simulink model "LAB4"  (R2025b)
settings: Solver=VariableStepAuto  StartTime=0.0  StopTime=20  RelTol=1e-3
libraries: simulink x1
settings Model: Creator=Wingshingsho  LastModifiedBy=Wingshingsho

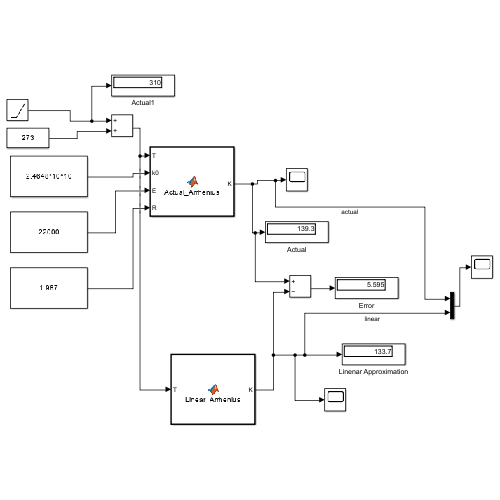
[thumbnail: Simulink's stored preview of the top-level diagram]
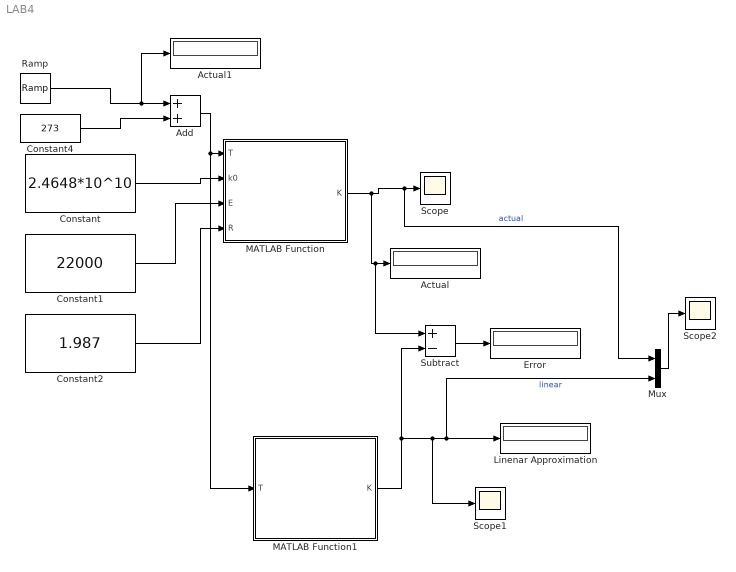
== system LAB4 ==
  Actual : Display
  Actual1 : Display
  Add : Sum
  Constant : Constant  Value=2.4648*10^10
  Constant1 : Constant  Value=22000
  Constant2 : Constant  Value=1.987
  Constant4 : Constant  Value=273
  Error : Display
  Linenar Approximation : Display
  MATLAB Function : MATLAB Function  TreatAsAtomicUnit=on
  MATLAB Function1 : MATLAB Function  TreatAsAtomicUnit=on
  Mux : Mux  Inputs=2
  Ramp : simulink/Sources/Ramp  slope=(310-290)/20  start=0  InitialOutput=290
  Scope : Scope
      settings: ActiveDisplayYMinimum=62.404399178444322  ActiveDisplayYMaximum=147.8382745404146
  Scope1 : Scope
      settings: ActiveDisplayYMinimum=-1  ActiveDisplayYMaximum=1
  Scope2 : Scope
      settings: ActiveDisplayYMinimum=57.175639124472795  ActiveDisplayYMaximum=148.41924787974477  DataLoggingVariableName=ScopeData2
  Subtract : Sum  Inputs=+-
  wires:
  Constant1/1 -> MATLAB Function/3(E)
  Constant/1 -> MATLAB Function/2(k0)
  Constant2/1 -> MATLAB Function/4(R)
  Constant4/1 -> Add/2
  Add/1 -> MATLAB Function1/1(T), MATLAB Function/1(T)
  MATLAB Function/1(K) -> Subtract/1, Actual/1, Mux/1, Scope/1  "actual"
  MATLAB Function1/1(K) -> Subtract/2, Scope1/1, Mux/2, Linenar Approximation/1  "linear"
  Subtract/1 -> Error/1
  Ramp/1 -> Actual1/1, Add/1
  Mux/1 -> Scope2/1

== matlab function LAB4/MATLAB Function1 ==
  data: T input; K output
function K = Linear_Arrhenius(T)

K = 100+3.37*(T-573);
end

== matlab function LAB4/MATLAB Function ==
  data: T input; K output; k0 input; E input; R input
function K = Actual_Arrhenius(T,k0,E,R)


K = k0*exp(-E/(R*T));
end
